simulink model "w2p3_model"  (R2020a)
settings: Solver=VariableStepAuto  StartTime=0.0  StopTime=120  RelTol=1e-3
model workspace (MAT data in the model file):
  Param = Simulink.Parameter
  Param.DataType = 'auto'
  Param.Dimensions = [0 0]
  b = Simulink.Parameter
  b.Value = 50
  b.DataType = 'auto'
  b.Dimensions = [1 1]
  kd = Simulink.Parameter
  kd.Value = 45
  kd.DataType = 'auto'
  kd.Dimensions = [1 1]
  ki = Simulink.Parameter
  ki.Value = 40
  ki.DataType = 'auto'
  ki.Dimensions = [1 1]
  kp = Simulink.Parameter
  kp.Value = 800
  kp.DataType = 'auto'
  kp.Dimensions = [1 1]
  m = Simulink.Parameter
  m.Value = 1000
  m.DataType = 'auto'
  m.Dimensions = [1 1]
  u = Simulink.Parameter
  u.Value = 500
  u.DataType = 'auto'
  u.Dimensions = [1 1]
settings Model: Creator=avn19  LastModifiedBy=avn19

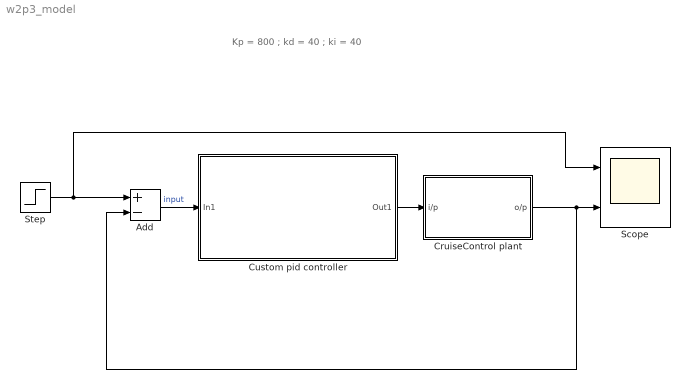
== system w2p3_model ==
  note: Kp = 800 ; kd = 40 ; ki = 40
  Add : Sum  Inputs=+-
  CruiseControl plant : Subsystem
  Custom pid controller : Subsystem
  Scope : Scope  NumInputPorts=2
  Step : Step  SampleTime=0
  wires:
  CruiseControl plant/1(o/p) -> Add/2, Scope/2
  Step/1 -> Scope/1, Add/1
  Add/1 -> Custom pid controller/1(In1)  "input"
  Custom pid controller/1(Out1) -> CruiseControl plant/1(i/p)

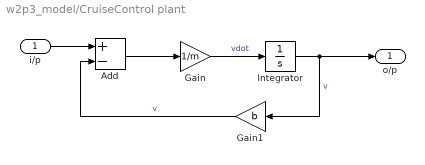
== system w2p3_model/CruiseControl plant ==
  i/p : Inport
  Add : Sum  Inputs=+-
  Gain : Gain  Gain=1/m
  Gain1 : Gain  Gain=b
  Integrator : Integrator
  o/p : Outport
  wires:
  i/p/1 -> Add/1
  Gain/1 -> Integrator/1  "vdot"
  Integrator/1 -> o/p/1, Gain1/1  "v"
  Add/1 -> Gain/1
  Gain1/1 -> Add/2  "v"

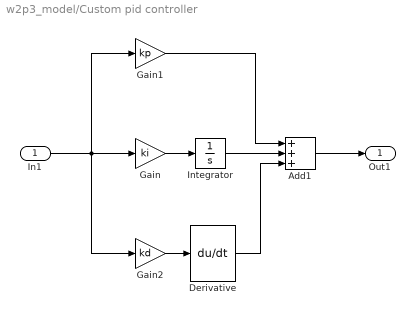
== system w2p3_model/Custom pid controller ==
  In1 : Inport
  Add1 : Sum  Inputs=+++
  Derivative : Derivative
  Gain : Gain  Gain=ki
  Gain1 : Gain  Gain=kp
  Gain2 : Gain  Gain=kd
  Integrator : Integrator
  Out1 : Outport
  wires:
  In1/1 -> Gain2/1, Gain/1, Gain1/1
  Derivative/1 -> Add1/3
  Gain2/1 -> Derivative/1
  Gain/1 -> Integrator/1
  Add1/1 -> Out1/1
  Gain1/1 -> Add1/1
  Integrator/1 -> Add1/2
